simulink model "s_pol4"  (Simulink 2.00)
settings: Solver=ode45  StartTime=0.0  StopTime=50  MaxStep=0.10  RelTol=1e-3  AbsTol=1e-6
values from neighbouring files (symbols this model uses):
  k1 = K(1)    [alqr1.m]    (also in alqrd1.m; apol1.m; pol1.m = -2*a*T1-1-T1/T2; pol2.m = -2*a*T1-1-T1/T2)
  k2 = K(2)    [alqr1.m]    (also in alqrd1.m; apol1.m; pol1.m = (a^2+b^2)*T1*T2-1-k1; pol2.m = (a^2+b^2)*T1*T2-1-k1)
  ki = 0.8/ks    [pol4.m]    (also in pol5.m = -Kn(n+1); pol7.m = -Kn(n+1))
  T1 = -5    [pol1.m]    (also in pol2.m; pol3.m; pol4.m)
  T2 = 10    [pol1.m]    (also in pol2.m; pol3.m; pol4.m)
settings Model: SaveTime=off  SaveOutput=off  ConsistencyChecking=off

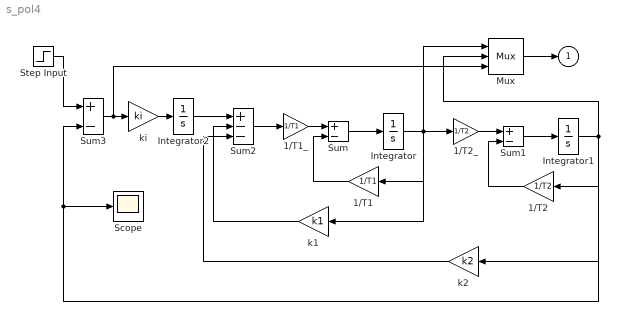
== system s_pol4 ==
  1/T1 : Gain  Orientation=left  Gain=1/T1
  1/T1_ : Gain  Gain=1/T1
  1/T2 : Gain  Orientation=left  Gain=1/T2
  1/T2_ : Gain  Gain=1/T2
  Integrator : Integrator  ExternalReset=none  InitialConditionSource=internal  InitialCondition=0  LimitOutput=off  UpperSaturationLimit=inf  LowerSaturationLimit=-inf  ShowSaturationPort=off  ShowStatePort=off  AbsoluteTolerance=auto
  Integrator1 : Integrator  ExternalReset=none  InitialConditionSource=internal  InitialCondition=0  LimitOutput=off  UpperSaturationLimit=inf  LowerSaturationLimit=-inf  ShowSaturationPort=off  ShowStatePort=off  AbsoluteTolerance=auto
  Integrator2 : Integrator  ExternalReset=none  InitialConditionSource=internal  InitialCondition=0  LimitOutput=off  UpperSaturationLimit=inf  LowerSaturationLimit=-inf  ShowSaturationPort=off  ShowStatePort=off  AbsoluteTolerance=auto
  Mux : Mux  Inputs=3
  Scope : Scope
      settings: TickLabels=on  TimeRange=50.000000  YMin=-1.540000  YMax=1.540000  SaveToWorkspace=off  SaveName=ScopeData
  Step Input : Step  Time=0  Before=0  After=1
  Sum : Sum  Inputs=+-
  Sum1 : Sum  Inputs=+-
  Sum2 : Sum  Inputs=+--
  Sum3 : Sum  Inputs=+-
  k1 : Gain  Orientation=left  Gain=k1
  k2 : Gain  Orientation=left  Gain=k2
  ki : Gain  Gain=ki
  " " : Outport  Port=1  InitialOutput=0
  wires:
  Sum3/1 -> Mux/3, ki/1
  Mux/1 -> " "/1
  Integrator2/1 -> Sum2/1
  ki/1 -> Integrator2/1
  k2/1 -> Sum2/3
  Step Input/1 -> Sum3/1
  k1/1 -> Sum2/2
  Integrator1/1 -> Mux/2, Scope/1, Sum3/2, k2/1, 1/T2/1
  Sum2/1 -> 1/T1_/1
  Integrator/1 -> Mux/1, k1/1, 1/T2_/1, 1/T1/1
  Sum1/1 -> Integrator1/1
  1/T2/1 -> Sum1/2
  1/T2_/1 -> Sum1/1
  Sum/1 -> Integrator/1
  1/T1/1 -> Sum/2
  1/T1_/1 -> Sum/1
